simulink model "project_345153"  (R2021a)
settings: Solver=ode45  StartTime=0  StopTime=StopTime  MaxStep=0.01  RelTol=1e-3  EnableMultiTasking=on
values from neighbouring files (symbols this model uses):
  p_des_x = [p_des_x, 0.8*dx]    [generateTrajectory.m]
  p_des_y = [p_des_y, 0.8*dy]    [generateTrajectory.m]
  p_des_z = [p_des_z, dz]    [generateTrajectory.m]
undefined symbols (not defined in the file or in its folder): Friction, Friction2, kd, ki, kk, kp, l1, l2, l3, m1, m2, m3, Normal, Normal2, p_act, p_des, Penetration, q_act, q_des, tau, X, Y, Z
libraries: sm_lib x40, Contact_Forces_Lib x26, nesl_utility x9, simulink x5, pid_lib x3
(part 2 of 2)

== matlab function project_345153/Direct kinematics1 ==
  data: q1 input; p output; q2 input; q3 input
function p = fcn(q1, q2, q3)
kk=5;
l1=kk*0.3;l2=kk*0.4;l3=kk*(0.4+0.2); % m
% direct kinematics
p = [-sin(q1)*(l3*cos(q2 + q3) + l2*cos(q2));...
 cos(q1)*(l3*cos(q2 + q3) + l2*cos(q2));...
      l1 + l3*sin(q2 + q3) + l2*sin(q2)-1];

== matlab function project_345153/q1 ==
  data: x input; q1 output; y input
function q1 = fcn(x,y)
q1 = atan2(y,x)-pi/2;
% q1 = atan2(y,x)+pi;
% As long as x,y \neq 0 both these solutions are valid
% When x,y = 0 the arm is in a singular configuration 
% and there are infinitely many possible solutions for q1.

== matlab function project_345153/q3 ==
  data: x input; q3 output; y input; z input; l1 input; l2 input; l3 input
function q3 = fcn(x,y,z,l1,l2,l3)
% D = (x^2 + y^2 + z^2 - l2^2 -l3^2)/(2*l_2*l_3);
% q3 = atan2(sqrt(1-D^2), D);
kk=5;
l3=l3+0.2;
l3=kk*l3;
l2=kk*l2;
argument = (l2^2+l3^2-x^2-y^2-(z)^2)/(2*l2*l3);
q3 = pi - acos(argument);

== matlab function project_345153/q2 ==
  data: x input; q2 output; y input; z input; l1 input; l2 input; l3 input
function q2 = fcn(x,y,z,l1,l2,l3)
% q2 = atan2(z, sqrt(x^2 + y^2)) - atan2(l3*sin(q3), l2+l3*cos(q3));
kk=5;
l3=l3+0.2;
l3=kk*l3;
l2=l2*kk;
argument = (x^2+y^2+z^2+l2^2-l3^2)/(2*sqrt(x^2+y^2+z^2)*l2);
alpha = acos(argument);
gamma = atan2(z, sqrt(x^2+y^2));
q2 = gamma - alpha;
